simulink model "tarea2"  (R2015a)
settings: Solver=ode45  StartTime=0.0  StopTime=20  RelTol=1e-3
settings Model: Creator=Alumnos  LastModifiedBy=Alumnos

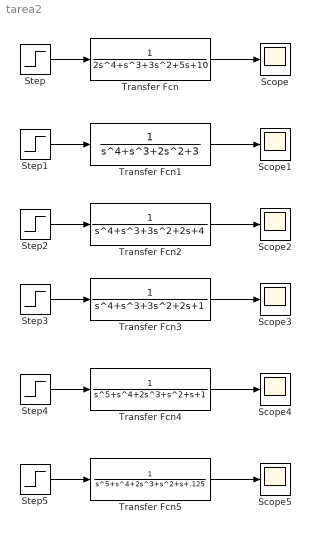
== system tarea2 ==
  Scope{,1..5} (6 alike) : Scope
      Scope2 settings: SaveName=ScopeData2
      Scope3 settings: SaveName=ScopeData3
      Scope4 settings: SaveName=ScopeData4
      Scope5 settings: SaveName=ScopeData5
  Step{,1..5} (6 alike) : Step  SampleTime=0
  Transfer Fcn : TransferFcn  Denominator=[2 1 3 5 10]
  Transfer Fcn1 : TransferFcn  Denominator=[1 1 2 0 3]
  Transfer Fcn2 : TransferFcn  Denominator=[1 1 3 2 4]
  Transfer Fcn3 : TransferFcn  Denominator=[1 1 3 2 1]
  Transfer Fcn4 : TransferFcn  Denominator=[1 1 2 1 1 1]
  Transfer Fcn5 : TransferFcn  Denominator=[1 1 2 1 1 .125]
  wires:
  Step/1 -> Transfer Fcn/1
  Transfer Fcn/1 -> Scope/1
  Step1/1 -> Transfer Fcn1/1
  Transfer Fcn1/1 -> Scope1/1
  Step2/1 -> Transfer Fcn2/1
  Transfer Fcn2/1 -> Scope2/1
  Step3/1 -> Transfer Fcn3/1
  Transfer Fcn3/1 -> Scope3/1
  Step4/1 -> Transfer Fcn4/1
  Transfer Fcn4/1 -> Scope4/1
  Step5/1 -> Transfer Fcn5/1
  Transfer Fcn5/1 -> Scope5/1
